simulink model "linear1_model"  (R2012b)
settings: Solver=ode45  StartTime=0.0  StopTime=10.0  RelTol=1e-3
settings Model: Creator=stsuei  LastModifiedBy=stsuei
settings DataIOCC: LimitDataPoints=off  LoadExternalInput=on
settings DebuggingCC: SolverPrmCheckMsg=none

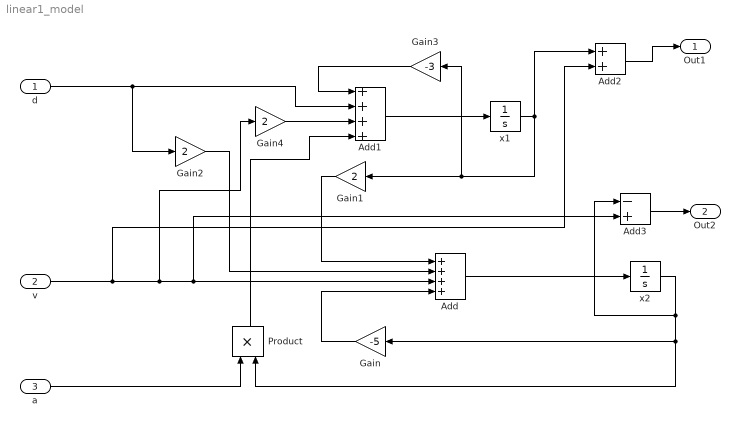
== system linear1_model ==
  d : Inport  PortDimensions=1
  v : Inport  Port=2  PortDimensions=1
  a : Inport  Port=3  PortDimensions=1
  Add : Sum  Inputs=++++
  Add1 : Sum  Inputs=++++
  Add2 : Sum
  Add3 : Sum  Inputs=-+
  Gain : Gain  Gain=-5
  Gain1 : Gain  Gain=2
  Gain2 : Gain  Gain=2
  Gain3 : Gain  Gain=-3
  Gain4 : Gain  Gain=2
  Product : Product  RndMeth=Zero
  x1 : Integrator
  x2 : Integrator
  Out1 : Outport
  Out2 : Outport  Port=2
  wires:
  x2/1 -> Add3/1, Product/2, Gain/1
  x1/1 -> Gain1/1, Gain3/1, Add2/1
  d/1 -> Gain2/1, Add1/2
  Add/1 -> x2/1
  Gain/1 -> Add/4
  Gain2/1 -> Add/2
  v/1 -> Add2/2, Add3/2, Add/3, Gain4/1
  Gain1/1 -> Add/1
  a/1 -> Product/1
  Add1/1 -> x1/1
  Product/1 -> Add1/4
  Gain4/1 -> Add1/3
  Gain3/1 -> Add1/1
  Add2/1 -> Out1/1
  Add3/1 -> Out2/1
